simulink model "flyback_dt"  (R2021b)
settings: Solver=FixedStepDiscrete  StartTime=0.0  StopTime=100e-3  RelTol=1e-3
undefined symbols (not defined in the file): DiscIntNeverNeededParam
Description:
  | Symmetric FIR Filter
  | This example shows how to use HDL Coder(TM) to check, generate,
  | and verify HDL for a fixed-point symmetric FIR filter.
settings Model: DataTypeOverride=Off  Creator=The MathWorks, Inc.  LastModifiedBy=Marco Milanesi
settings SolverCC: AlgebraicLoopSolver=TrustRegion  AutoInsertRateTranBlk=on
settings DataIOCC: LimitDataPoints=on  SaveFormat=Array  SaveOutput=off  SignalLogging=off  SaveTime=off  ReturnWorkspaceOutputs=off  SignalLoggingName=logsOut
settings OptimizationCC: BlockReduction=off  BooleanDataType=off  ConditionallyExecuteInputs=off  DefaultParameterBehavior=Inlined  InheritOutputTypeSmallerThanSingle=on  InlineInvariantSignals=on  ExpressionDepthLimit=2147483647  InitFltsAndDblsToZero=on  LifeSpan=inf  BufferReusableBoundary=off
settings DebuggingCC: AlgebraicLoopMsg=error  SaveWithParameterizedLinksMsg=none  UnderspecifiedInitializationDetection=Classic  MergeDetectMultiDrivingBlocksExec=none  CheckExecutionContextPreStartOutputMsg=on  SignalResolutionControl=TryResolveAllWithWarning  MultiTaskDSMMsg=warning  MultiTaskCondExecSysMsg=none  SingleTaskRateTransMsg=error  IntegerOverflowMsg=none  ParameterPrecisionLossMsg=none  FcnCallInpInsideContextMsg=warning  BusObjectLabelMismatch=none  StateNameClashWarn=warning  SFUnexpectedBacktrackingDiag=warning  SFNoUnconditionalDefaultTransitionDiag=warning  SFExecutionAtInitializationDiag=none  SFMachineParentedDataDiag=warning  IntegerSaturationMsg=none  ArithmeticOperatorsInVariantConditions=warning
settings HardwareCC: ProdBitPerPointer=32  ProdBitPerSizeT=32  ProdBitPerPtrDiffT=32  ProdLargestAtomicFloat=None  ProdIntDivRoundTo=Undefined  ProdEndianess=Unspecified  ProdWordSize=32  ProdHWDeviceType=ASIC/FPGA  TargetUnknown=on  ProdEqTarget=off
settings ModelReferenceCC: PropagateSignalLabelsOutOfModel=off
settings SFSimCC: SimUseLocalCustomCode=off  CustomCodeUndefinedFunction=UseInterfaceOnly
settings RTWCC: RTWUseLocalCustomCode=off
settings CodeAppCC: StateflowObjectComments=on
settings GRTTargetCC: TargetFcnLib=ansi_tfl_tmw.mat  TargetLangStandard=C89/C90 (ANSI)  CombineOutputUpdateFcns=off  GRTInterface=on
settings ConfigComp: CovMetricSettings=dw  CovSaveCumulativeToWorkspaceVar=on  CovSaveSingleToWorkspaceVar=on  CovExternalEMLEnable=off

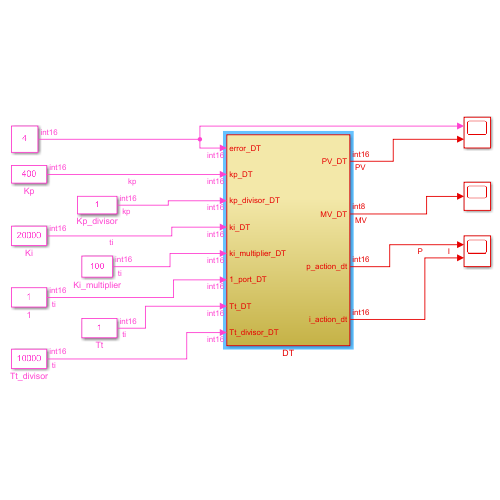
[thumbnail: Simulink's stored preview of the top-level diagram]
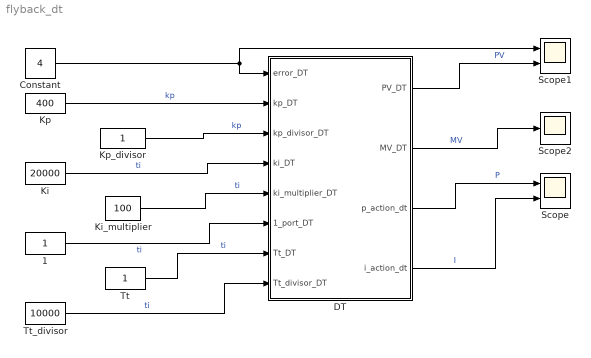
== system flyback_dt ==
  1 : Constant  OutDataTypeStr=fixdt(1,16,0)
  Constant : Constant  Value=4  OutDataTypeStr=fixdt(1,16,0)
  DT : Subsystem
  Ki : Constant  Value=20000  OutDataTypeStr=fixdt(1,16,0)
  Ki_multiplier : Constant  Value=100  OutDataTypeStr=fixdt(1,16,0)
  Kp : Constant  Value=400  OutDataTypeStr=fixdt(1,16,0)
  Kp_divisor : Constant  OutDataTypeStr=fixdt(1,16,0)
  Scope : Scope  NumInputPorts=2
  Scope1 : Scope  NumInputPorts=2
  Scope2 : Scope
  Tt : Constant  OutDataTypeStr=fixdt(1,16,0)
  Tt_divisor : Constant  Value=10000  OutDataTypeStr=fixdt(1,16,0)
  wires:
  Constant/1 -> DT/1(error_DT), Scope1/1
  DT/3(p_action_dt) -> Scope/1  "P"
  DT/1(PV_DT) -> Scope1/2  "PV"
  DT/2(MV_DT) -> Scope2/1  "MV"
  DT/4(i_action_dt) -> Scope/2  "I"
  Ki_multiplier/1 -> DT/5(ki_multiplier_DT)  "ti"
  Kp/1 -> DT/2(kp_DT)  "kp"
  Tt_divisor/1 -> DT/8(Tt_divisor_DT)  "ti"
  Ki/1 -> DT/4(ki_DT)  "ti"
  1/1 -> DT/6(1_port_DT)  "ti"
  Kp_divisor/1 -> DT/3(kp_divisor_DT)  "kp"
  Tt/1 -> DT/7(Tt_DT)  "ti"

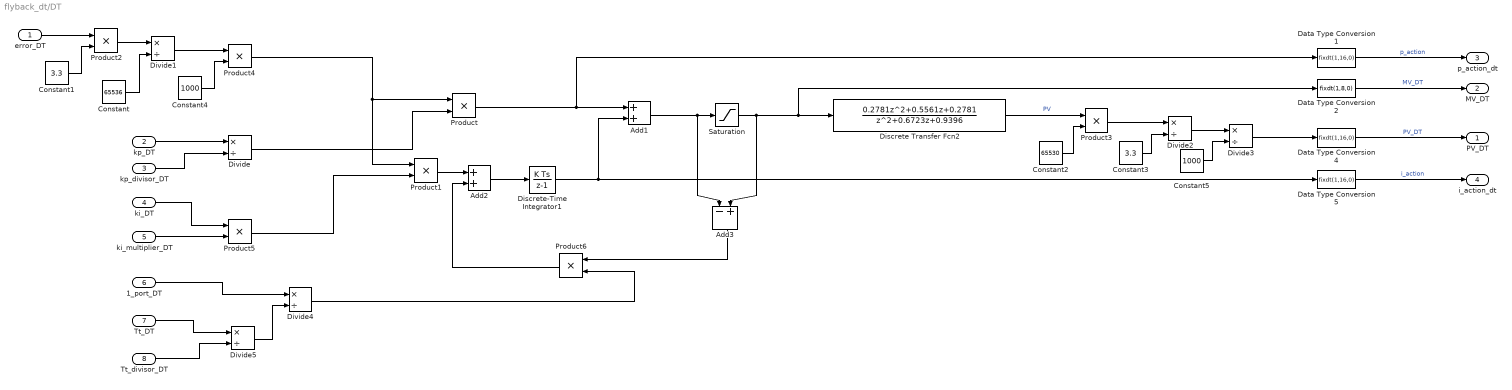
== system flyback_dt/DT ==
  error_DT : Inport  OutDataTypeStr=fixdt(1,16,0)  SampleTime=80e-9
  kp_DT : Inport  Port=2  OutDataTypeStr=fixdt(1,16,0)  SampleTime=80e-9
  kp_divisor_DT : Inport  Port=3  OutDataTypeStr=fixdt(1,16,0)  SampleTime=80e-9
  ki_DT : Inport  Port=4  OutDataTypeStr=fixdt(1,16,0)  SampleTime=80e-9
  ki_multiplier_DT : Inport  Port=5  OutDataTypeStr=fixdt(1,16,0)  SampleTime=80e-9
  1_port_DT : Inport  Port=6  OutDataTypeStr=fixdt(1,16,0)  SampleTime=80e-9
  Tt_DT : Inport  Port=7  OutDataTypeStr=fixdt(1,16,0)  SampleTime=80e-9
  Tt_divisor_DT : Inport  Port=8  OutDataTypeStr=fixdt(1,16,0)  SampleTime=80e-9
  Add1 : Sum  AccumDataTypeStr=fixdt(1,16,0)  OutDataTypeStr=fixdt(1,16,0)
  Add2 : Sum  AccumDataTypeStr=fixdt(1,16,0)  OutDataTypeStr=fixdt(1,16,0)
  Add3 : Sum  Inputs=-+  AccumDataTypeStr=fixdt(1,16,0)  OutDataTypeStr=fixdt(1,16,0)
  Constant : Constant  Value=65536  OutDataTypeStr=fixdt(1,32,0)  SampleTime=80e-9
  Constant1 : Constant  Value=3.3  OutDataTypeStr=fixdt(1,16,0)  SampleTime=80e-9
  Constant2 : Constant  Value=65530  OutDataTypeStr=fixdt(1,32,0)  SampleTime=80e-9
  Constant3 : Constant  Value=3.3  OutDataTypeStr=fixdt(1,16,0)  SampleTime=80e-9
  Constant4 : Constant  Value=1000  OutDataTypeStr=fixdt(1,16,0)  SampleTime=80e-9
  Constant5 : Constant  Value=1000  OutDataTypeStr=fixdt(1,16,0)  SampleTime=80e-9
  Data Type Conversion1 : DataTypeConversion  OutDataTypeStr=fixdt(1,16,0)
  Data Type Conversion2 : DataTypeConversion  OutDataTypeStr=fixdt(1,8,0)
  Data Type Conversion4 : DataTypeConversion  OutDataTypeStr=fixdt(1,16,0)
  Data Type Conversion5 : DataTypeConversion  OutDataTypeStr=fixdt(1,16,0)
  Discrete Transfer Fcn2 : DiscreteTransferFcn  Numerator=[0.2781 0.5561 0.2781]  Denominator=[1 0.6723 0.9396]  SampleTime=80e-9  NumCoefDataTypeStr=fixdt(1,16,0)  DenCoefDataTypeStr=fixdt(1,16,0)  NumProductDataTypeStr=fixdt(1,16,0)  DenProductDataTypeStr=fixdt(1,16,0)  NumAccumDataTypeStr=fixdt(1,16,0)  DenAccumDataTypeStr=fixdt(1,16,0)  OutDataTypeStr=fixdt(1,16,0)
  Discrete-Time Integrator1 : DiscreteIntegrator  SampleTime=80e-9  OutDataTypeStr=fixdt(1,16,0)  ICPrevOutput=DiscIntNeverNeededParam  ICPrevScaledInput=DiscIntNeverNeededParam
  Divide{,1..5} (6 alike) : Product  Inputs=*/  OutDataTypeStr=fixdt(1,16,0)  RndMeth=Zero  SaturateOnIntegerOverflow=on
  Product{,1..6} (7 alike) : Product  OutDataTypeStr=fixdt(1,16,0)
  Saturation : Saturate  UpperLimit=255  LowerLimit=0  OutDataTypeStr=fixdt(1,16,0)
  PV_DT : Outport  OutDataTypeStr=fixdt(1,16,0)  SampleTime=80e-9  VectorParamsAs1DForOutWhenUnconnected=off
  MV_DT : Outport  Port=2  OutDataTypeStr=fixdt(1,8,0)  SampleTime=80e-9  VectorParamsAs1DForOutWhenUnconnected=off
  p_action_dt : Outport  Port=3  OutDataTypeStr=fixdt(1,16,0)  SampleTime=80e-9  VectorParamsAs1DForOutWhenUnconnected=off
  i_action_dt : Outport  Port=4  OutDataTypeStr=fixdt(1,16,0)  SampleTime=80e-9  VectorParamsAs1DForOutWhenUnconnected=off
  wires:
  Discrete Transfer Fcn2/1 -> Product3/1  "PV"
  Data Type Conversion1/1 -> p_action_dt/1  "p_action"
  Data Type Conversion2/1 -> MV_DT/1  "MV_DT"
  Data Type Conversion4/1 -> PV_DT/1  "PV_DT"
  Data Type Conversion5/1 -> i_action_dt/1  "i_action"
  error_DT/1 -> Product2/1
  Product2/1 -> Divide1/1
  Constant/1 -> Divide1/2
  Constant1/1 -> Product2/2
  Product3/1 -> Divide2/1
  Constant2/1 -> Product3/2
  Constant3/1 -> Divide2/2
  Constant4/1 -> Product4/2
  Divide1/1 -> Product4/1
  Constant5/1 -> Divide3/2
  Divide2/1 -> Divide3/1
  Divide3/1 -> Data Type Conversion4/1
  Tt_DT/1 -> Divide5/1
  Add2/1 -> Discrete-Time Integrator1/1
  Product1/1 -> Add2/1
  Divide5/1 -> Divide4/2
  Tt_divisor_DT/1 -> Divide5/2
  Divide/1 -> Product/2
  Product/1 -> Data Type Conversion1/1, Add1/1
  1_port_DT/1 -> Divide4/1
  kp_divisor_DT/1 -> Divide/2
  Saturation/1 -> Data Type Conversion2/1, Discrete Transfer Fcn2/1, Add3/2
  Product4/1 -> Product/1, Product1/1
  Product6/1 -> Add2/2
  kp_DT/1 -> Divide/1
  ki_multiplier_DT/1 -> Product5/2
  Add3/1 -> Product6/1
  Discrete-Time Integrator1/1 -> Add1/2, Data Type Conversion5/1
  Divide4/1 -> Product6/2
  Product5/1 -> Product1/2
  ki_DT/1 -> Product5/1
  Add1/1 -> Saturation/1, Add3/1
